simulink model "Pendubot"  (Simulink 10.3)
settings: Solver=ode45  StartTime=0.0  StopTime=8  RelTol=1e-3  AbsTol=1e-4
values from neighbouring files (symbols this model uses):
  Ts = 0.004    [Pendubot_ini.m]
undefined symbols (not defined in the file or in its folder): pendubot_eqt, pendubot_reg
libraries: simulink x2
Description:
  | Non-linear mathematical model of pendubot electro-mechanical system (underactuated pendulum system).
settings Model: Creator=Hynek Prochazka  LastModifiedBy=Colin  ExtModeTrigMode=oneshot  ExtModeArmWhenConnect=off
settings SolverCC: AutoScaleAbsTol=off
settings DataIOCC: SaveOutput=off
settings OptimizationCC: BlockReduction=off  BooleanDataType=off
settings DebuggingCC: SaveWithParameterizedLinksMsg=none  SignalResolutionControl=TryResolveAllWithWarning  MultiTaskDSMMsg=warning  MultiTaskCondExecSysMsg=none
settings HardwareCC: TargetUnknown=on
settings RTWCC: TemplateMakefile=grt_unix.tmf
settings ConfigComp: CovSFcnEnable=off

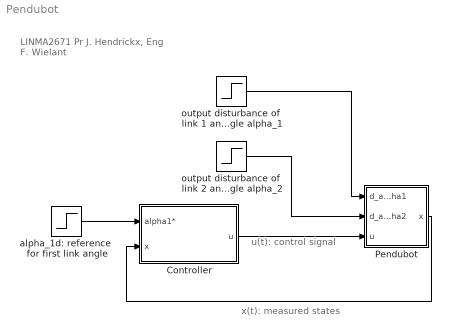
== system Pendubot ==
  note: u(t):
      | control signal
  note: x(t): measured states
  note: LINMA2671
      | Pr J. Hendrickx, Eng F. Wielant
  Controller : Subsystem
  Pendubot : Subsystem  mask(Pendubot){x10=pi, x20=0, x30=pi, x40=0, Ts=Ts}
      mask prompts: x10 "Initial angle of link 1:"; x20 "Initial angular speed for link 1 :"; x30 "Initial angle of link 2 :"; x40 "Initial angular speed for link 2 :"; Ts "Sampling time [s] :"
      mask help: Initial conditions (initial state)
      mask Display:
      | plot(0.1*[1 9],0.1*[1 1])
      | plot(0.1*[1.5 1.5 8.5 8.5],0.1*[1 4 4 1])
      | plot(0.1*[5.2 8.2],0.1*[1 5])
      | plot(0.1*[4.8 7.8],0.1*[1 5])
      | plot(0.1*[7.8 5.8],0.1*[5 9.5])
      | plot(0.1*[8.2 6.2],0.1*[5 9.5])
  "alpha_1d: reference  for first link angle " : Step  Time=2  Before=pi  After=4*pi/5  SampleTime=Ts
  output disturbance of  link 1 angle alpha_1 : Step  Time=5  After=0.2  SampleTime=Ts
  output disturbance of  link 2 angle alpha_2 : Step  Time=2  After=0.1  SampleTime=Ts
  wires:
  output disturbance of  link 1 angle alpha_1/1 -> Pendubot/1(d_alpha1)
  Pendubot/1(x) -> Controller/2(x)
  "alpha_1d: reference  for first link angle "/1 -> Controller/1(alpha1*)
  Controller/1(u) -> Pendubot/3(u)
  output disturbance of  link 2 angle alpha_2/1 -> Pendubot/2(d_alpha2)

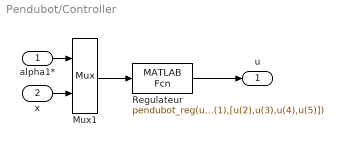
== system Pendubot/Controller ==
  alpha1* : Inport
  x : Inport  Port=2
  Mux1 : Mux  Inputs=2
  Regulateur : MATLABFcn  MATLABFcn=pendubot_reg(u(1),[u(2),u(3),u(4),u(5)])
  u : Outport
  wires:
  alpha1*/1 -> Mux1/1
  x/1 -> Mux1/2
  Mux1/1 -> Regulateur/1
  Regulateur/1 -> u/1

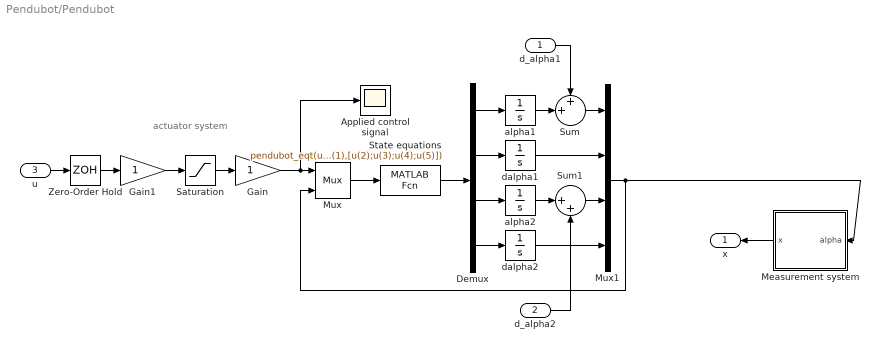
== system Pendubot/Pendubot ==
  note: actuator system
  d_alpha1 : Inport
  d_alpha2 : Inport  Port=2
  u : Inport  Port=3
  Applied control signal : Scope
  Demux : Demux
      settings: DisplayOption=none
  Gain : Gain  SaturateOnIntegerOverflow=on  OutDataTypeStr=Inherit: Same as input  ParamDataTypeStr=Inherit: Same as input
  Gain1 : Gain  SaturateOnIntegerOverflow=on  OutDataTypeStr=Inherit: Same as input  ParamDataTypeStr=Inherit: Same as input
  Measurement system : Subsystem
  Mux : Mux  Inputs=2
  Mux1 : Mux
  Saturation : Saturate  UpperLimit=10  LowerLimit=-10
  State equations : MATLABFcn  MATLABFcn=pendubot_eqt(u(1),[u(2);u(3);u(4);u(5)])  OutputDimensions=4
  Sum : Sum  Inputs=++|  InputSameDT=on  SaturateOnIntegerOverflow=on  OutDataTypeStr=Inherit: Same as first input
  Sum1 : Sum  Inputs=|++  InputSameDT=on  SaturateOnIntegerOverflow=on  OutDataTypeStr=Inherit: Same as first input
  Zero-Order Hold : ZeroOrderHold  SampleTime=Ts
  alpha1 : Integrator  InitialCondition=x10
  alpha2 : Integrator  InitialCondition=x30
  dalpha1 : Integrator  InitialCondition=x20
  dalpha2 : Integrator  InitialCondition=x40
  x : Outport
  wires:
  u/1 -> Zero-Order Hold/1
  State equations/1 -> Demux/1
  Mux/1 -> State equations/1
  Saturation/1 -> Gain/1
  Zero-Order Hold/1 -> Gain1/1
  Gain1/1 -> Saturation/1
  Gain/1 -> Mux/1, Applied control signal/1
  Mux1/1 -> Mux/2, Measurement system/1(alpha)
  dalpha2/1 -> Mux1/4
  Demux/1 -> alpha1/1
  Demux/2 -> dalpha1/1
  Demux/3 -> alpha2/1
  Demux/4 -> dalpha2/1
  Sum/1 -> Mux1/1
  Sum1/1 -> Mux1/3
  dalpha1/1 -> Mux1/2
  alpha1/1 -> Sum/2
  d_alpha1/1 -> Sum/1
  alpha2/1 -> Sum1/1
  d_alpha2/1 -> Sum1/2
  Measurement system/1(x) -> x/1

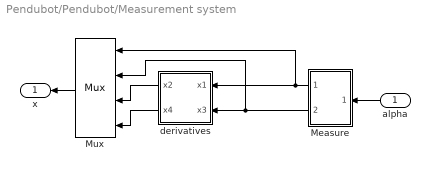
== system Pendubot/Pendubot/Measurement system ==
  alpha : Inport
  Measure : Subsystem
  Mux : Mux
  derivatives : Subsystem
  x : Outport
  wires:
  derivatives/2(x4) -> Mux/4
  Mux/1 -> x/1
  Measure/1(xm(1)) -> derivatives/1(x1), Mux/1
  alpha/1 -> Measure/1(alpha)
  Measure/2(xm(1)1) -> derivatives/2(x3), Mux/2
  derivatives/1(x2) -> Mux/3

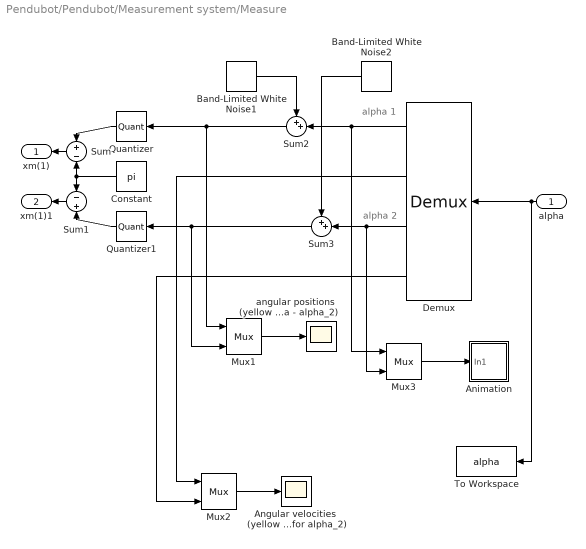
== system Pendubot/Pendubot/Measurement system/Measure ==
  note: alpha 1
  note: alpha 2
  alpha : Inport
  "Angular velocities  (yellow - for alpha_1,  magenta - for alpha_2) " : Scope
  Animation : Subsystem  mask(Animation Block){ts=10*0.003}
      mask prompts: ts "Sample time:"
      mask Display: plot([.1,.9],[.9,.9],[.5,.2],[.9,.25],[.475,.475,.525,.525,.475],[.875,.925,.925,.875,.875])
  Band-Limited White Noise1 : simulink/Sources/Band-Limited White Noise  Cov=[1e-8]  Ts=Ts  seed=[23341]
  Band-Limited White Noise2 : simulink/Sources/Band-Limited White Noise  Cov=[1e-7]  Ts=Ts  seed=[32214]
  Constant : Constant  Value=pi
  Demux : Demux
      settings: DisplayOption=none
  Mux1 : Mux  Inputs=2
  Mux2 : Mux  Inputs=2
  Mux3 : Mux  Inputs=2
  Quantizer : Quantizer  QuantizationInterval=2*pi/5000
  Quantizer1 : Quantizer  QuantizationInterval=2*pi/5000
  Sum : Sum  Inputs=+-  InputSameDT=on  SaturateOnIntegerOverflow=on  OutDataTypeStr=Inherit: Same as first input
  Sum1 : Sum  Inputs=-+  InputSameDT=on  SaturateOnIntegerOverflow=on  OutDataTypeStr=Inherit: Same as first input
  Sum2 : Sum  Inputs=++|  InputSameDT=on  SaturateOnIntegerOverflow=on  OutDataTypeStr=Inherit: Same as first input
  Sum3 : Sum  Inputs=++|  InputSameDT=on  SaturateOnIntegerOverflow=on  OutDataTypeStr=Inherit: Same as first input
  To Workspace : ToWorkspace  VariableName=alpha  SampleTime=Ts
  "angular positions  (yellow - alpha_1,  magenta - alpha_2)" : Scope
  xm(1) : Outport  Tag=alpha1
  xm(1)1 : Outport  Port=2
  wires:
  alpha/1 -> To Workspace/1, Demux/1
  Demux/2 -> Mux2/1
  Demux/4 -> Mux2/2
  Mux2/1 -> "Angular velocities  (yellow - for alpha_1,  magenta - for alpha_2) "/1
  Sum/1 -> xm(1)/1
  Quantizer/1 -> Sum/1
  Sum1/1 -> xm(1)1/1
  Quantizer1/1 -> Sum1/2
  Constant/1 -> Sum/2, Sum1/1
  Band-Limited White Noise1/1 -> Sum2/1
  Band-Limited White Noise2/1 -> Sum3/1
  Sum2/1 -> Quantizer/1, Mux1/1
  Sum3/1 -> Quantizer1/1, Mux1/2
  Mux1/1 -> "angular positions  (yellow - alpha_1,  magenta - alpha_2)"/1
  Demux/1 -> Sum2/2, Mux3/1
  Demux/3 -> Sum3/2, Mux3/2
  Mux3/1 -> Animation/1(In1)

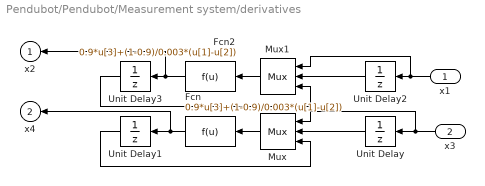
== system Pendubot/Pendubot/Measurement system/derivatives ==
  x1 : Inport
  x3 : Inport  Port=2
  Fcn : Fcn  Expr=0.9*u[3]+(1-0.9)/0.003*(u[1]-u[2])
  Fcn2 : Fcn  Expr=0.9*u[3]+(1-0.9)/0.003*(u[1]-u[2])
  Mux : Mux  Inputs=3
  Mux1 : Mux  Inputs=3
  Unit Delay{,1..3} (4 alike) : UnitDelay  SampleTime=Ts  HasFrameUpgradeWarning=on
  x2 : Outport
  x4 : Outport  Port=2
  wires:
  Unit Delay/1 -> Mux/2
  Mux/1 -> Fcn/1
  Unit Delay1/1 -> Mux/3
  Fcn/1 -> Unit Delay1/1, x4/1
  x3/1 -> Unit Delay/1, Mux/1
  Unit Delay2/1 -> Mux1/2
  Mux1/1 -> Fcn2/1
  Unit Delay3/1 -> Mux1/3
  x1/1 -> Unit Delay2/1, Mux1/1
  Fcn2/1 -> Unit Delay3/1, x2/1

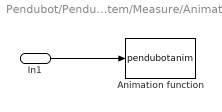
== system Pendubot/Pendubot/Measurement system/Measure/Animation ==
  In1 : Inport
  Animation function : S-Function  FunctionName=pendubotanim  Parameters=ts  SFunctionDeploymentMode=off  EnableBusSupport=off
      settings: DeleteFcn=if ~isempty(findobj('type','figure','name','simppend Animation'));close('simppend Animation'); end;
  wires:
  In1/1 -> Animation function/1
